simulink model "EngineDynamometer"  (R2025b)
settings: configuration reference "EngDynoVariable" (kept outside this file)
model workspace (MAT data in the model file):
  DynOperatingPts : timeseries (value not decoded)
undefined symbols (not defined in the file): CiDynoMaxTurboSpd, CiDynoSSSpdCmd, CiDynoSSTrqCmd, DynoResultsBlock, EnvAbsPrs, EnvAirTemp, EnvRair, ExhCamPhaseCmd, InjPw, IntkCamPhaseCmd, Line, PlntEngAfrStoich, PlntEngCps, PlntEngNCyl, PlntEngSinj, PlntEngVd, si, si0, SiDynoMaxTurboSpd, SiDynoOpenLoopEngSpdCmdPts, SiDynoOpenLoopExhCamPhsCmdPts, SiDynoOpenLoopIntCamPhsCmdPts, SiDynoOpenLoopLambdaCmdPts, SiDynoOpenLoopMaxMAP, SiDynoOpenLoopSpkDeltaCmdPts, SiDynoOpenLoopSteadyStateWaitLimit, SiDynoOpenLoopTpCmdPts, SiDynoOpenLoopWAPCmdPts, SiDynoSSSpdCmd, SiDynoSSTrqCmd, SiDynoSSWaitLim, SpkAdv, ThrPosPctCmd, WgAreaPctCmd
libraries: autolibutils x4, autolibpowerinfoutils x1, simulink x1
(part 2 of 3)

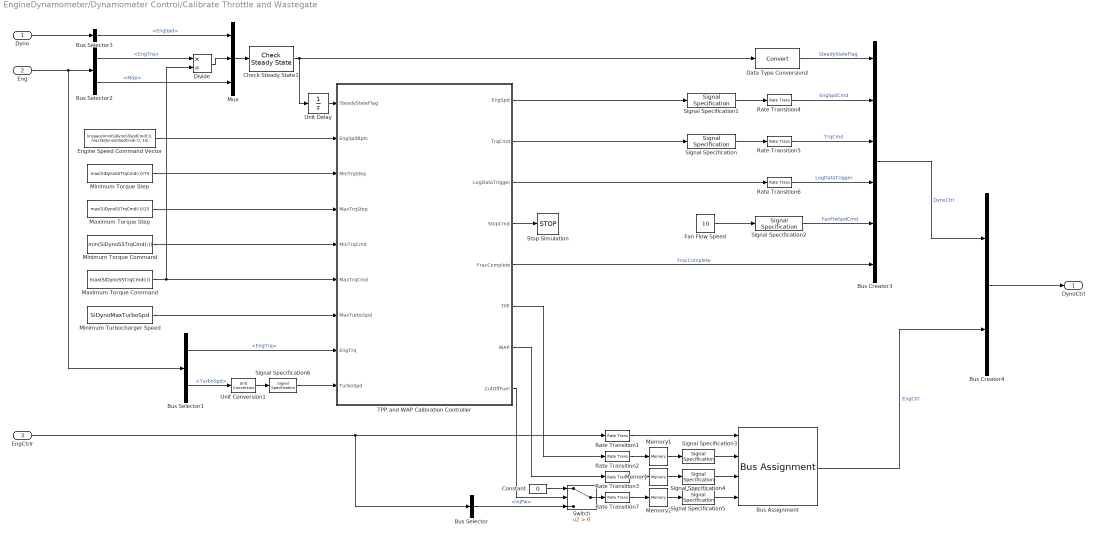
== system EngineDynamometer/Dynamometer Control/Calibrate Throttle and Wastegate ==
  Dyno : Inport
  Eng : Inport  Port=2
  EngCtrlr : Inport  Port=3
  Bus Assignment : BusAssignment  AssignedSignals=ThrPosPctCmd,WgAreaPctCmd,InjPw
  Bus Creator3 : BusCreator  Inputs=6
  Bus Creator4 : BusCreator  Inputs=2
  Bus Selector : BusSelector  OutputSignals=InjPw
  Bus Selector1 : BusSelector  OutputSignals=EngPlnt.EngTrq,EngPlnt.TurboSpd
  Bus Selector2 : BusSelector  OutputSignals=EngPlnt.EngTrq,EngPlnt.Map
  Bus Selector3 : BusSelector  OutputSignals=DynoPlnt.EngSpd
  Check Steady State1 : autolibutils/Check Steady State  N=4  F=50  Ts=0.2  SteadyThresh=[0.1; 0.003; 2500]  HoldTime=0.5  aMode=aMode
  Constant : Constant  Value=0
  Data Type Conversion2 : DataTypeConversion  SaturateOnIntegerOverflow=off  RndMeth=Floor
  Divide : Product  Inputs=*/
  Engine Speed Command Vector : Constant  Value=linspace(min(SiDynoSSSpdCmd(:)), max(SiDynoSSSpdCmd(:)), 15)
  Fan Flow Speed : Constant  Value=10
  Maximum Torque Command : Constant  Value=max(SiDynoSSTrqCmd(:))
  Maximum Torque Step : Constant  Value=max(SiDynoSSTrqCmd(:))/25
  Memory : Memory  InitialCondition=100
  Memory1 : Memory
  Memory2 : Memory  InitialCondition=100
  Minimum Torque Command : Constant  Value=min(SiDynoSSTrqCmd(:))
  Minimum Torque Step : Constant  Value=max(SiDynoSSTrqCmd(:))/75
  Minimum Turbocharger Speed : Constant  Value=SiDynoMaxTurboSpd
  Mux : Mux  Inputs=3
  Rate Transition{1..3,7} (4 alike) : RateTransition  Deterministic=off  OutPortSampleTimeOpt=Inherit
  Rate Transition4 : RateTransition  Deterministic=off
  Rate Transition5 : RateTransition  Deterministic=off
  Rate Transition6 : RateTransition  Deterministic=off
  Signal Specification : SignalSpecification  Unit=N*m
  Signal Specification1 : SignalSpecification  Unit=rpm
  Signal Specification2 : SignalSpecification  Unit=N*m
  Signal Specification3 : SignalSpecification  Unit=%
  Signal Specification4 : SignalSpecification  Unit=%
  Signal Specification5 : SignalSpecification  Unit=ms
  Signal Specification6 : SignalSpecification  Unit=rpm
  Stop Simulation : Stop
  Switch : Switch  Criteria=u2 > Threshold  SaturateOnIntegerOverflow=off  InputSameDT=off
  TPP and WAP Calibration Controller : Stateflow chart  TreatAsAtomicUnit=on
  Unit Conversion1 : UnitConversion
  Unit Delay : UnitDelay  SampleTime=-1  HasFrameUpgradeWarning=on
  DynoCtrl : Outport  VectorParamsAs1DForOutWhenUnconnected=off
  wires:
  Divide/1 -> Mux/2
  Bus Selector3/1 -> Mux/1  "<EngSpd>"
  Bus Selector2/1 -> Divide/1  "<EngTrq>"
  TPP and WAP Calibration Controller/2(TrqCmd) -> Signal Specification/1
  Bus Selector2/2 -> Mux/3  "<Map>"
  TPP and WAP Calibration Controller/7(WAP) -> Rate Transition3/1
  TPP and WAP Calibration Controller/6(TPP) -> Rate Transition2/1
  Bus Creator3/1 -> Bus Creator4/1  "DynoCtrl"
  Bus Creator4/1 -> DynoCtrl/1
  Mux/1 -> Check Steady State1/1
  Data Type Conversion2/1 -> Bus Creator3/1  "SteadyStateFlag"
  Rate Transition6/1 -> Bus Creator3/4  "LogDataTrigger"
  Rate Transition5/1 -> Bus Creator3/3  "TrqCmd"
  Rate Transition4/1 -> Bus Creator3/2  "EngSpdCmd"
  Fan Flow Speed/1 -> Signal Specification2/1
  Maximum Torque Step/1 -> TPP and WAP Calibration Controller/4(MaxTrqStep)
  Engine Speed Command Vector/1 -> TPP and WAP Calibration Controller/2(EngSpdBpts)
  TPP and WAP Calibration Controller/4(StopCmd) -> Stop Simulation/1
  Dyno/1 -> Bus Selector3/1
  Eng/1 -> Bus Selector1/1, Bus Selector2/1
  Rate Transition3/1 -> Memory/1
  Rate Transition2/1 -> Memory1/1
  Bus Selector1/1 -> TPP and WAP Calibration Controller/8(EngTrq)  "<EngTrq>"
  Bus Selector1/2 -> Unit Conversion1/1  "<TurboSpd>"
  Signal Specification/1 -> Rate Transition5/1
  Signal Specification1/1 -> Rate Transition4/1
  TPP and WAP Calibration Controller/1(EngSpd) -> Signal Specification1/1
  Signal Specification2/1 -> Bus Creator3/5  "FanFlwSpdCmd"
  TPP and WAP Calibration Controller/5(FracComplete) -> Bus Creator3/6  "FracComplete"
  EngCtrlr/1 -> Rate Transition1/1, Bus Selector/1
  Memory/1 -> Signal Specification4/1
  Memory1/1 -> Signal Specification3/1
  Bus Assignment/1 -> Bus Creator4/2  "EngCtrl"
  Signal Specification3/1 -> Bus Assignment/2
  Signal Specification4/1 -> Bus Assignment/3
  Rate Transition1/1 -> Bus Assignment/1
  Minimum Torque Step/1 -> TPP and WAP Calibration Controller/3(MinTrqStep)
  Minimum Torque Command/1 -> TPP and WAP Calibration Controller/5(MinTrqCmd)
  Maximum Torque Command/1 -> Divide/2, TPP and WAP Calibration Controller/6(MaxTrqCmd)
  Check Steady State1/1 -> Unit Delay/1, Data Type Conversion2/1
  TPP and WAP Calibration Controller/3(LogDataTrigger) -> Rate Transition6/1
  Minimum Turbocharger Speed/1 -> TPP and WAP Calibration Controller/7(MaxTurboSpd)
  Unit Conversion1/1 -> Signal Specification6/1
  Signal Specification6/1 -> TPP and WAP Calibration Controller/9(TurboSpd)
  Memory2/1 -> Signal Specification5/1
  Rate Transition7/1 -> Memory2/1
  Signal Specification5/1 -> Bus Assignment/4
  Switch/1 -> Rate Transition7/1
  TPP and WAP Calibration Controller/8(CutOffFuel) -> Switch/2
  Constant/1 -> Switch/1
  Bus Selector/1 -> Switch/3  "<InjPw>"
  Unit Delay/1 -> TPP and WAP Calibration Controller/1(SteadyStateFlag)

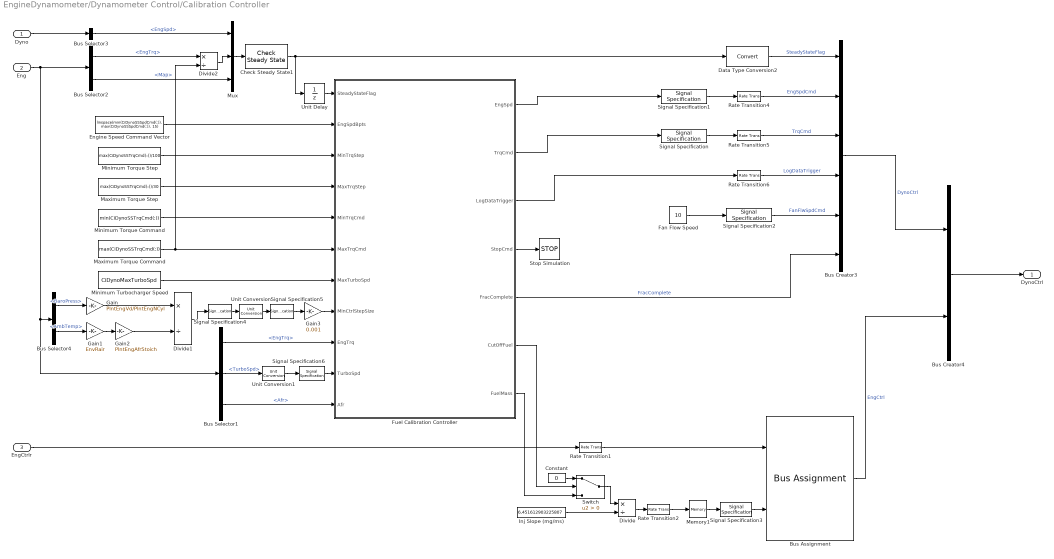
== system EngineDynamometer/Dynamometer Control/Calibration Controller ==
  Dyno : Inport
  Eng : Inport  Port=2
  EngCtrlr : Inport  Port=3
  Bus Assignment : BusAssignment  AssignedSignals=InjPw
  Bus Creator3 : BusCreator  Inputs=6
  Bus Creator4 : BusCreator  Inputs=2
  Bus Selector1 : BusSelector  OutputSignals=EngPlnt.EngTrq,EngPlnt.TurboSpd,EngPlnt.Afr
  Bus Selector2 : BusSelector  OutputSignals=EngPlnt.EngTrq,EngPlnt.Map
  Bus Selector3 : BusSelector  OutputSignals=DynoPlnt.EngSpd
  Bus Selector4 : BusSelector  OutputSignals=Env.BaroPress,Env.AmbTemp
  Check Steady State1 : autolibutils/Check Steady State  N=4  F=25  Ts=0.1  SteadyThresh=[0.1; 0.002; 500]  HoldTime=0.5  aMode=aMode
  Constant : Constant  Value=0
  Data Type Conversion2 : DataTypeConversion  SaturateOnIntegerOverflow=off  RndMeth=Floor
  Divide : Product  Inputs=*/
  Divide1 : Product  Inputs=*/
  Divide2 : Product  Inputs=*/
  Engine Speed Command Vector : Constant  Value=linspace(min(CiDynoSSSpdCmd(:)), max(CiDynoSSSpdCmd(:)), 15)
  Fan Flow Speed : Constant  Value=10
  Fuel Calibration Controller : Stateflow chart  TreatAsAtomicUnit=on
  Gain : Gain  Gain=PlntEngVd/PlntEngNCyl
  Gain1 : Gain  Gain=EnvRair
  Gain2 : Gain  Gain=PlntEngAfrStoich
  Gain3 : Gain  Gain=0.001
  Inj Slope (mg/ms) : Constant  Value=6.451612903225807
  Maximum Torque Command : Constant  Value=max(CiDynoSSTrqCmd(:))
  Maximum Torque Step : Constant  Value=max(CiDynoSSTrqCmd(:))/30
  Memory1 : Memory
  Minimum Torque Command : Constant  Value=min(CiDynoSSTrqCmd(:))
  Minimum Torque Step : Constant  Value=max(CiDynoSSTrqCmd(:))/100
  Minimum Turbocharger Speed : Constant  Value=CiDynoMaxTurboSpd
  Mux : Mux  Inputs=3
  Rate Transition1 : RateTransition  Deterministic=off  OutPortSampleTimeOpt=Inherit
  Rate Transition2 : RateTransition  Deterministic=off  OutPortSampleTimeOpt=Inherit
  Rate Transition4 : RateTransition  Deterministic=off
  Rate Transition5 : RateTransition  Deterministic=off
  Rate Transition6 : RateTransition  Deterministic=off
  Signal Specification : SignalSpecification  Unit=N*m
  Signal Specification1 : SignalSpecification  Unit=rpm
  Signal Specification2 : SignalSpecification  Unit=N*m
  Signal Specification3 : SignalSpecification  Unit=ms
  Signal Specification4 : SignalSpecification  Unit=kg
  Signal Specification5 : SignalSpecification  Unit=mg
  Signal Specification6 : SignalSpecification  Unit=rpm
  Stop Simulation : Stop
  Switch : Switch  Criteria=u2 > Threshold  SaturateOnIntegerOverflow=off  InputSameDT=off
  Unit Conversion : UnitConversion
  Unit Conversion1 : UnitConversion
  Unit Delay : UnitDelay  SampleTime=-1  HasFrameUpgradeWarning=on
  DynoCtrl : Outport  VectorParamsAs1DForOutWhenUnconnected=off
  wires:
  Signal Specification5/1 -> Gain3/1
  Gain3/1 -> Fuel Calibration Controller/8(MinCtrlStepSize)
  Unit Conversion/1 -> Signal Specification5/1
  Divide1/1 -> Signal Specification4/1
  Signal Specification4/1 -> Unit Conversion/1
  Gain2/1 -> Divide1/2
  Gain/1 -> Divide1/1
  Gain1/1 -> Gain2/1
  Bus Selector4/1 -> Gain/1  "<BaroPress>"
  Bus Selector4/2 -> Gain1/1  "<AmbTemp>"
  Bus Selector3/1 -> Mux/1  "<EngSpd>"
  Bus Selector2/1 -> Divide2/1  "<EngTrq>"
  Fuel Calibration Controller/2(TrqCmd) -> Signal Specification/1
  Bus Selector2/2 -> Mux/3  "<Map>"
  Bus Creator3/1 -> Bus Creator4/1  "DynoCtrl"
  Bus Creator4/1 -> DynoCtrl/1
  Mux/1 -> Check Steady State1/1
  Data Type Conversion2/1 -> Bus Creator3/1  "SteadyStateFlag"
  Rate Transition6/1 -> Bus Creator3/4  "LogDataTrigger"
  Rate Transition5/1 -> Bus Creator3/3  "TrqCmd"
  Rate Transition4/1 -> Bus Creator3/2  "EngSpdCmd"
  Fan Flow Speed/1 -> Signal Specification2/1
  Maximum Torque Step/1 -> Fuel Calibration Controller/4(MaxTrqStep)
  Engine Speed Command Vector/1 -> Fuel Calibration Controller/2(EngSpdBpts)
  Fuel Calibration Controller/4(StopCmd) -> Stop Simulation/1
  Dyno/1 -> Bus Selector3/1
  Eng/1 -> Bus Selector4/1, Bus Selector1/1, Bus Selector2/1
  Rate Transition2/1 -> Memory1/1
  Bus Selector1/1 -> Fuel Calibration Controller/9(EngTrq)  "<EngTrq>"
  Bus Selector1/2 -> Unit Conversion1/1  "<TurboSpd>"
  Signal Specification/1 -> Rate Transition5/1
  Signal Specification1/1 -> Rate Transition4/1
  Fuel Calibration Controller/1(EngSpd) -> Signal Specification1/1
  Signal Specification2/1 -> Bus Creator3/5  "FanFlwSpdCmd"
  Fuel Calibration Controller/5(FracComplete) -> Bus Creator3/6  "FracComplete"
  EngCtrlr/1 -> Rate Transition1/1
  Memory1/1 -> Signal Specification3/1
  Bus Assignment/1 -> Bus Creator4/2  "EngCtrl"
  Signal Specification3/1 -> Bus Assignment/2
  Rate Transition1/1 -> Bus Assignment/1
  Minimum Torque Step/1 -> Fuel Calibration Controller/3(MinTrqStep)
  Minimum Torque Command/1 -> Fuel Calibration Controller/5(MinTrqCmd)
  Check Steady State1/1 -> Data Type Conversion2/1, Unit Delay/1
  Fuel Calibration Controller/3(LogDataTrigger) -> Rate Transition6/1
  Bus Selector1/3 -> Fuel Calibration Controller/11(Afr)  "<Afr>"
  Inj Slope (mg/ms)/1 -> Divide/2
  Divide/1 -> Rate Transition2/1
  Divide2/1 -> Mux/2
  Maximum Torque Command/1 -> Fuel Calibration Controller/6(MaxTrqCmd), Divide2/2
  Minimum Turbocharger Speed/1 -> Fuel Calibration Controller/7(MaxTurboSpd)
  Unit Conversion1/1 -> Signal Specification6/1
  Signal Specification6/1 -> Fuel Calibration Controller/10(TurboSpd)
  Constant/1 -> Switch/1
  Fuel Calibration Controller/6(CutOffFuel) -> Switch/2
  Switch/1 -> Divide/1
  Fuel Calibration Controller/7(FuelMass) -> Switch/3
  Unit Delay/1 -> Fuel Calibration Controller/1(SteadyStateFlag)

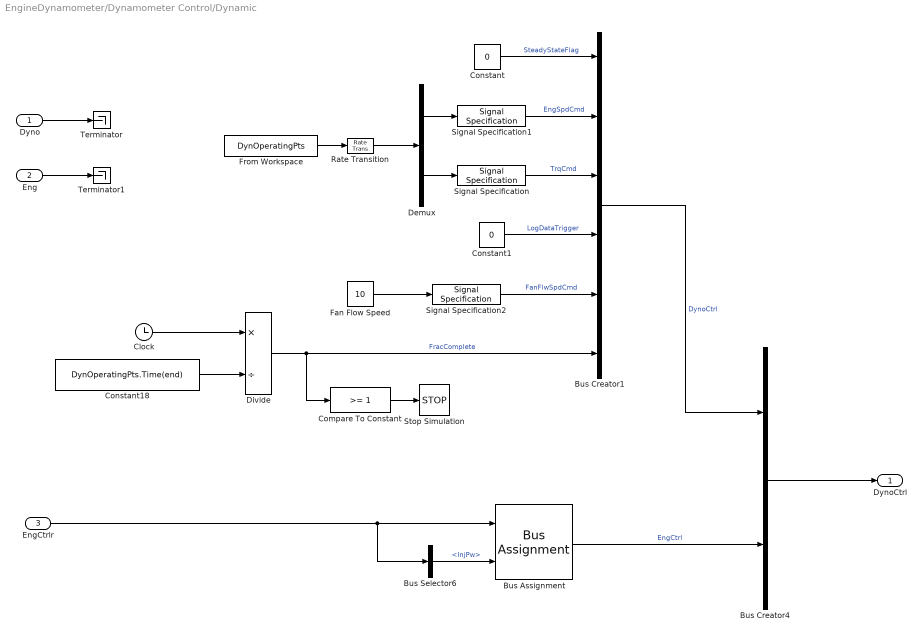
== system EngineDynamometer/Dynamometer Control/Dynamic ==
  Dyno : Inport
  Eng : Inport  Port=2
  EngCtrlr : Inport  Port=3
  Bus Assignment : BusAssignment  AssignedSignals=InjPw
  Bus Creator1 : BusCreator  Inputs=6
  Bus Creator4 : BusCreator  Inputs=2
  Bus Selector6 : BusSelector  OutputSignals=InjPw
  Clock : Clock
  Compare To Constant : simulink/Logic and Bit Operations/Compare To Constant  relop=>=  const=1  OutDataTypeStr=boolean
  Constant : Constant  Value=0
  Constant1 : Constant  Value=0
  Constant18 : Constant  Value=DynOperatingPts.Time(end)
  Demux : Demux  Outputs=2
  Divide : Product  Inputs=*/
  Fan Flow Speed : Constant  Value=10
  From Workspace : FromWorkspace  VariableName=DynOperatingPts  SampleTime=0.01  ZeroCross=off  OutputAfterFinalValue=Holding final value
  Rate Transition : RateTransition
  Signal Specification : SignalSpecification  Unit=N*m
  Signal Specification1 : SignalSpecification  Unit=rpm
  Signal Specification2 : SignalSpecification  Unit=m/s
  Stop Simulation : Stop
  Terminator : Terminator
  Terminator1 : Terminator
  DynoCtrl : Outport  VectorParamsAs1DForOutWhenUnconnected=off
  wires:
  Bus Creator1/1 -> Bus Creator4/1  "DynoCtrl"
  Bus Creator4/1 -> DynoCtrl/1
  Constant1/1 -> Bus Creator1/4  "LogDataTrigger"
  Constant/1 -> Bus Creator1/1  "SteadyStateFlag"
  Dyno/1 -> Terminator/1
  Demux/1 -> Signal Specification1/1
  Demux/2 -> Signal Specification/1
  Clock/1 -> Divide/1
  Compare To Constant/1 -> Stop Simulation/1
  From Workspace/1 -> Rate Transition/1
  Rate Transition/1 -> Demux/1
  Fan Flow Speed/1 -> Signal Specification2/1
  Signal Specification2/1 -> Bus Creator1/5  "FanFlwSpdCmd"
  Signal Specification1/1 -> Bus Creator1/2  "EngSpdCmd"
  Signal Specification/1 -> Bus Creator1/3  "TrqCmd"
  Divide/1 -> Compare To Constant/1, Bus Creator1/6  "FracComplete"
  Constant18/1 -> Divide/2
  EngCtrlr/1 -> Bus Assignment/1, Bus Selector6/1
  Bus Assignment/1 -> Bus Creator4/2  "EngCtrl"
  Bus Selector6/1 -> Bus Assignment/2  "<InjPw>"
  Eng/1 -> Terminator1/1

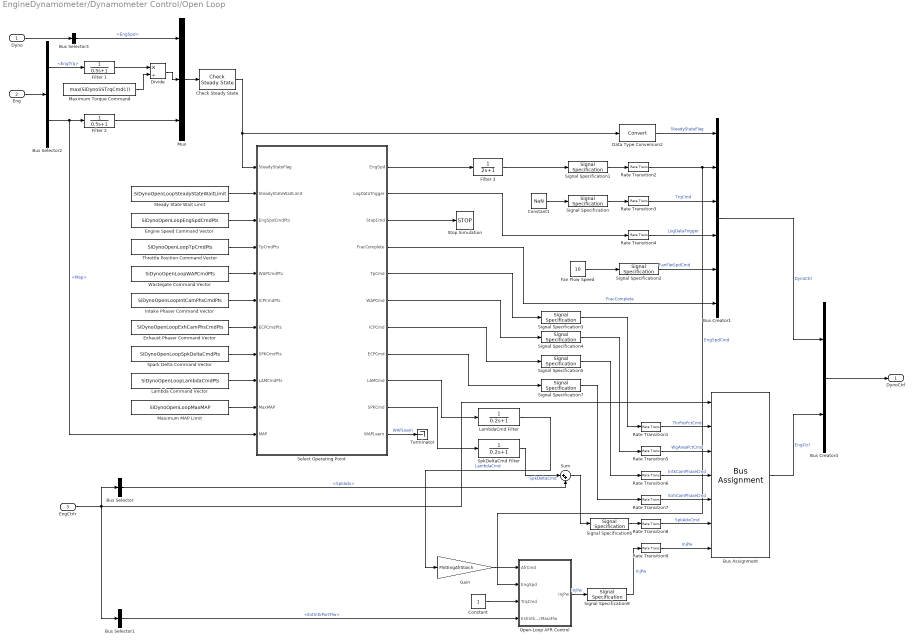
== system EngineDynamometer/Dynamometer Control/Open Loop ==
  Dyno : Inport
  Eng : Inport  Port=2
  EngCtrlr : Inport  Port=3
  Bus Assignment : BusAssignment  AssignedSignals=ThrPosPctCmd,WgAreaPctCmd,IntkCamPhaseCmd,ExhCamPhaseCmd,SpkAdv,InjPw
  Bus Creator1 : BusCreator  Inputs=6
  Bus Creator4 : BusCreator  Inputs=2
  Bus Selector : BusSelector  OutputSignals=SpkAdv
  Bus Selector1 : BusSelector  OutputSignals=EstIntkPortFlw
  Bus Selector2 : BusSelector  OutputSignals=EngPlnt.EngTrq,EngPlnt.Map
  Bus Selector3 : BusSelector  OutputSignals=DynoPlnt.EngSpd
  Check Steady State : autolibutils/Check Steady State  N=4  F=25  Ts=0.1  SteadyThresh=[0.25; 0.002; 2000]  HoldTime=1  aMode=aMode
  Constant : Constant
  Constant1 : Constant  Value=NaN
  Data Type Conversion2 : DataTypeConversion  SaturateOnIntegerOverflow=off  RndMeth=Floor
  Divide : Product  Inputs=*/
  Engine Speed Command Vector : Constant  Value=SiDynoOpenLoopEngSpdCmdPts
  Exhaust Phaser Command Vector : Constant  Value=SiDynoOpenLoopExhCamPhsCmdPts
  Fan Flow Speed : Constant  Value=10
  Filter 1 : TransferFcn  Denominator=[0.5 1]
  Filter 2 : TransferFcn  Denominator=[0.5 1]
  Filter 3 : TransferFcn  Denominator=[2 1]
  Gain : Gain  Gain=PlntEngAfrStoich
  Intake Phaser Command Vector : Constant  Value=SiDynoOpenLoopIntCamPhsCmdPts
  Lambda Command Vector : Constant  Value=SiDynoOpenLoopLambdaCmdPts
  LambdaCmd Filter : TransferFcn  Denominator=[0.2 1]
  Maximum MAP Limit : Constant  Value=SiDynoOpenLoopMaxMAP
  Maximum Torque Command : Constant  Value=max(SiDynoSSTrqCmd(:))
  Mux : Mux  Inputs=3
  Open-Loop AFR Control : Subsystem
      settings: LibrarySourceBlock=autolibengctrlr/SI Controller/Controllers/Fuel/Open-Loop AFR Control
  Rate Transition{1..9} (9 alike) : RateTransition
  Select Operating Point : Stateflow chart  TreatAsAtomicUnit=on
      settings: PortSchema="{\"entries\":[{\"content\":{\"sides\":[{\"content\":{\"connectorIds\":[\"In1\",\"In2\",\"In3\",\"In4\",\"In5\",\"In6\",\"In7\",\"In8\",\"In9\",\"In11\",\"In10\"]},\"type\":\"ConnectorPlacement.EquallySpacedRectSide\",\"uuid\":\"1175ad6d-9dc6-48de-a8de-c94bf62b3e4b\"},{\"content\":{\"connectorIds\":[\"Out1\",\"Out2\",\"Out3\",\"Out4\",\"Out5\",\"Out6\",\"Out7\",\"Out8\",\"Out9\",\"Out10\",\"Out11\"],\"side\":\"RIGHT\"},\"type\":\"ConnectorPlacement.EquallySpacedRectSide\",\"uuid\":\"1be9bb31-04dd-492d-b81f-3e8c0fe512b8\"},{\"content\":{\"connectorIds\":[],\"side\":\"TOP\"},\"type\":\"ConnectorPlacement.EquallySpacedRectSide\",\"uuid\":\"9ff59bc2-c566-4c7d-a042-0eeecf9e5d1c\"}]},\"type\":\"ConnectorPlacement.EquallySpacedConnector\",\"uuid\":\"78b64ed8-c9b9-4ccc-b3ba-c3246a70f380\"}],\"packageUris\":[\"http://schema.mathworks.com/mf0/Connector/R2020b\"],\"version\":\"1.0\"}"
  Signal Specification : SignalSpecification  Unit=N*m
  Signal Specification1 : SignalSpecification  Unit=rpm
  Signal Specification2 : SignalSpecification  Unit=m/s
  Signal Specification3 : SignalSpecification  Unit=%
  Signal Specification4 : SignalSpecification  Unit=%
  Signal Specification5 : SignalSpecification  Unit=deg
  Signal Specification6 : SignalSpecification  Unit=deg
  Signal Specification7 : SignalSpecification  Unit=deg
  Signal Specification8 : SignalSpecification  Unit=ms
  Spark Delta Command Vector : Constant  Value=SiDynoOpenLoopSpkDeltaCmdPts
  SpkDeltaCmd Filter : TransferFcn  Denominator=[0.2 1]
  Steady State Wait Limit : Constant  Value=SiDynoOpenLoopSteadyStateWaitLimit
  Stop Simulation : Stop
  Sum : Sum  Inputs=|++
  Terminator : Terminator
  Throttle Position Command Vector : Constant  Value=SiDynoOpenLoopTpCmdPts
  Wastegate Command Vector : Constant  Value=SiDynoOpenLoopWAPCmdPts
  DynoCtrl : Outport  VectorParamsAs1DForOutWhenUnconnected=off
  wires:
  Maximum Torque Command/1 -> Divide/2
  Divide/1 -> Mux/2
  Select Operating Point/4(FracComplete) -> Bus Creator1/6  "FracComplete"
  Signal Specification/1 -> Rate Transition3/1
  Signal Specification1/1 -> Rate Transition2/1
  Signal Specification2/1 -> Bus Creator1/5  "FanFlwSpdCmd"
  Fan Flow Speed/1 -> Signal Specification2/1
  Engine Speed Command Vector/1 -> Select Operating Point/3(EngSpdCmdPts)
  Throttle Position Command Vector/1 -> Select Operating Point/4(TpCmdPts)
  Select Operating Point/2(LogDataTrigger) -> Rate Transition4/1
  Rate Transition2/1 -> Open-Loop AFR Control/2(EngSpd), Bus Creator1/2  "EngSpdCmd"
  Rate Transition3/1 -> Bus Creator1/3  "TrqCmd"
  Rate Transition4/1 -> Bus Creator1/4  "LogDataTrigger"
  Data Type Conversion2/1 -> Bus Creator1/1  "SteadyStateFlag"
  Check Steady State/1 -> Data Type Conversion2/1, Select Operating Point/1(SteadyStateFlag)
  Bus Creator4/1 -> DynoCtrl/1
  Bus Creator1/1 -> Bus Creator4/1  "DynoCtrl"
  Bus Assignment/1 -> Bus Creator4/2  "EngCtrl"
  Eng/1 -> Bus Selector2/1
  Dyno/1 -> Bus Selector3/1
  Mux/1 -> Check Steady State/1
  Bus Selector3/1 -> Mux/1  "<EngSpd>"
  EngCtrlr/1 -> Bus Selector1/1, Bus Selector/1, Bus Assignment/1
  Steady State Wait Limit/1 -> Select Operating Point/2(SteadyStateWaitLimit)
  Bus Selector2/1 -> Filter 1/1  "<EngTrq>"
  Filter 1/1 -> Divide/1
  Bus Selector2/2 -> Select Operating Point/10(MAP), Filter 2/1  "<Map>"
  Filter 2/1 -> Mux/3
  Filter 3/1 -> Signal Specification1/1
  Wastegate Command Vector/1 -> Select Operating Point/5(WAPCmdPts)
  Rate Transition1/1 -> Bus Assignment/2  "ThrPosPctCmd"
  Select Operating Point/5(TpCmd) -> Signal Specification3/1
  Select Operating Point/6(WAPCmd) -> Signal Specification4/1
  Rate Transition5/1 -> Bus Assignment/3  "WgAreaPctCmd"
  Select Operating Point/1(EngSpd) -> Filter 3/1
  Select Operating Point/3(StopCmd) -> Stop Simulation/1
  Intake Phaser Command Vector/1 -> Select Operating Point/6(ICPCmdPts)
  Exhaust Phaser Command Vector/1 -> Select Operating Point/7(ECPCmdPts)
  Signal Specification5/1 -> Rate Transition6/1
  Signal Specification7/1 -> Rate Transition7/1
  Select Operating Point/7(ICPCmd) -> Signal Specification5/1
  Select Operating Point/8(ECPCmd) -> Signal Specification7/1
  Rate Transition7/1 -> Bus Assignment/5  "ExhCamPhaseCmd"
  Rate Transition6/1 -> Bus Assignment/4  "IntkCamPhaseCmd"
  Spark Delta Command Vector/1 -> Select Operating Point/8(SPKCmdPts)
  Lambda Command Vector/1 -> Select Operating Point/9(LAMCmdPts)
  Select Operating Point/9(LAMCmd) -> LambdaCmd Filter/1
  Bus Selector/1 -> Sum/2  "<SpkAdv>"
  Sum/1 -> Signal Specification6/1
  Rate Transition8/1 -> Bus Assignment/6  "SpkAdvCmd"
  Signal Specification6/1 -> Rate Transition8/1
  LambdaCmd Filter/1 -> Gain/1  "LambdaCmd"
  SpkDeltaCmd Filter/1 -> Sum/1  "SpkDeltaCmd"
  Select Operating Point/10(SPKCmd) -> SpkDeltaCmd Filter/1
  Gain/1 -> Open-Loop AFR Control/1(AfrCmd)
  Constant/1 -> Open-Loop AFR Control/3(TrqCmd)
  Rate Transition9/1 -> Bus Assignment/7  "InjPw"
  Open-Loop AFR Control/1(InjPw) -> Signal Specification8/1  "InjPw"
  Signal Specification8/1 -> Rate Transition9/1  "InjPw"
  Bus Selector1/1 -> Open-Loop AFR Control/4(EstIntkAirMassFlw)  "<EstIntkPortFlw>"
  Signal Specification3/1 -> Rate Transition1/1
  Signal Specification4/1 -> Rate Transition5/1
  Maximum MAP Limit/1 -> Select Operating Point/11(MaxMAP)
  Select Operating Point/11(WAPLearn) -> Terminator/1  "WAPLearn"
  Constant1/1 -> Signal Specification/1

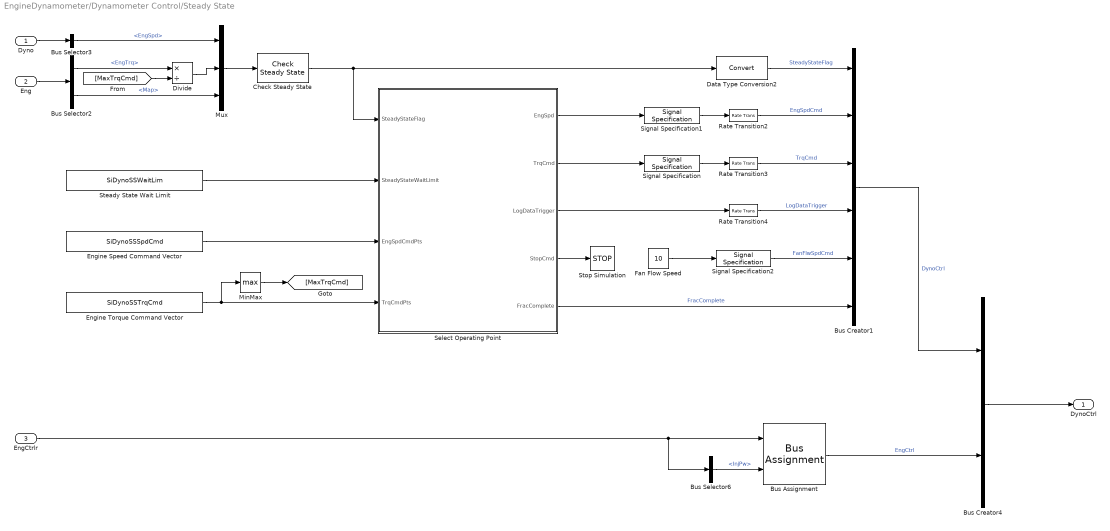
== system EngineDynamometer/Dynamometer Control/Steady State ==
  Dyno : Inport
  Eng : Inport  Port=2
  EngCtrlr : Inport  Port=3
  Bus Assignment : BusAssignment  AssignedSignals=InjPw
  Bus Creator1 : BusCreator  Inputs=6
  Bus Creator4 : BusCreator  Inputs=2
  Bus Selector2 : BusSelector  OutputSignals=EngPlnt.EngTrq,EngPlnt.Map
  Bus Selector3 : BusSelector  OutputSignals=DynoPlnt.EngSpd
  Bus Selector6 : BusSelector  OutputSignals=InjPw
  Check Steady State : autolibutils/Check Steady State  N=4  F=25  Ts=0.1  SteadyThresh=[0.25; 0.002; 2000]  HoldTime=1  aMode=aMode
  Data Type Conversion2 : DataTypeConversion  SaturateOnIntegerOverflow=off  RndMeth=Floor
  Divide : Product  Inputs=*/
  Engine Speed Command Vector : Constant  Value=SiDynoSSSpdCmd
  Engine Torque Command Vector : Constant  Value=SiDynoSSTrqCmd
  Fan Flow Speed : Constant  Value=10
  MinMax : MinMax  Function=max
  Mux : Mux  Inputs=3
  Rate Transition2 : RateTransition
  Rate Transition3 : RateTransition
  Rate Transition4 : RateTransition
  Select Operating Point : Stateflow chart  TreatAsAtomicUnit=on
  Signal Specification : SignalSpecification  Unit=N*m
  Signal Specification1 : SignalSpecification  Unit=rpm
  Signal Specification2 : SignalSpecification  Unit=m/s
  Steady State Wait Limit : Constant  Value=SiDynoSSWaitLim
  Stop Simulation : Stop
  DynoCtrl : Outport  VectorParamsAs1DForOutWhenUnconnected=off
  wires:
  Divide/1 -> Mux/2
  Select Operating Point/5(FracComplete) -> Bus Creator1/6  "FracComplete"
  Signal Specification/1 -> Rate Transition3/1
  Signal Specification1/1 -> Rate Transition2/1
  Signal Specification2/1 -> Bus Creator1/5  "FanFlwSpdCmd"
  Fan Flow Speed/1 -> Signal Specification2/1
  Select Operating Point/4(StopCmd) -> Stop Simulation/1
  Engine Speed Command Vector/1 -> Select Operating Point/3(EngSpdCmdPts)
  Engine Torque Command Vector/1 -> MinMax/1, Select Operating Point/4(TrqCmdPts)
  Select Operating Point/1(EngSpd) -> Signal Specification1/1
  Select Operating Point/2(TrqCmd) -> Signal Specification/1
  Select Operating Point/3(LogDataTrigger) -> Rate Transition4/1
  Rate Transition2/1 -> Bus Creator1/2  "EngSpdCmd"
  Rate Transition3/1 -> Bus Creator1/3  "TrqCmd"
  Rate Transition4/1 -> Bus Creator1/4  "LogDataTrigger"
  Data Type Conversion2/1 -> Bus Creator1/1  "SteadyStateFlag"
  Check Steady State/1 -> Select Operating Point/1(SteadyStateFlag), Data Type Conversion2/1
  Bus Creator4/1 -> DynoCtrl/1
  Bus Creator1/1 -> Bus Creator4/1  "DynoCtrl"
  Bus Assignment/1 -> Bus Creator4/2  "EngCtrl"
  Eng/1 -> Bus Selector2/1
  Dyno/1 -> Bus Selector3/1
  Mux/1 -> Check Steady State/1
  Bus Selector2/2 -> Mux/3  "<Map>"
  Bus Selector2/1 -> Divide/1  "<EngTrq>"
  Bus Selector3/1 -> Mux/1  "<EngSpd>"
  EngCtrlr/1 -> Bus Selector6/1, Bus Assignment/1
  Bus Selector6/1 -> Bus Assignment/2  "<InjPw>"
  Steady State Wait Limit/1 -> Select Operating Point/2(SteadyStateWaitLimit)
  MinMax/1 -> [MaxTrqCmd]
  [MaxTrqCmd] -> Divide/2

== system EngineDynamometer/Engine System/Dynamometer Engine Control ==
  Dyno : Inport
  Bus Selector : BusSelector  OutputSignals=DynoCtrl.EngCtrl
  Ctrl : Outport  VectorParamsAs1DForOutWhenUnconnected=off
  wires:
  Dyno/1 -> Bus Selector/1
  Bus Selector/1 -> Ctrl/1  "<EngCtrl>"

== system EngineDynamometer/Engine System/Engine Controller ==
  Env : Inport
  Dyno : Inport  Port=2
  EngPlnt : Inport  Port=3
  Engine Control : Subsystem  Variant=on  VariantControlMode=label  VariantControl=Choice  LabelModeActiveChoice=SI Engine Controller
  Engine Control Input : Subsystem
  Engine Control Output : Subsystem
  EngCtrlrOutput : Outport  VectorParamsAs1DForOutWhenUnconnected=off
  wires:
  Engine Control Output/1(EngCtrlrOutput) -> EngCtrlrOutput/1
  Dyno/1 -> Engine Control Input/1(Dyno)
  Env/1 -> Engine Control Input/2(Env)
  EngPlnt/1 -> Engine Control Input/3(VehPlnt)
  Engine Control Input/1(TrqCmd) -> Engine Control/1(TrqCmd)
  Engine Control Input/2(EngSpd) -> Engine Control/2(EngSpd)
  Engine Control Input/3(Map) -> Engine Control/3(Map)
  Engine Control Input/4(Mat) -> Engine Control/4(Mat)
  Engine Control Input/5(ThrPosPct) -> Engine Control/5(ThrPosPct)
  Engine Control Input/6(WgAreaPct) -> Engine Control/6(WgAreaPct)
  Engine Control Input/7(IntkCamPhase) -> Engine Control/7(IntkCamPhase)
  Engine Control Input/8(ExhCamPhase) -> Engine Control/8(ExhCamPhase)
  Engine Control Input/9(TurboRackPos) -> Engine Control/9(TurboRackPos)
  Engine Control Input/10(EgrVlvAreaPct) -> Engine Control/10(EgrVlvAreaPct)
  Engine Control Input/11(VarCompRatioPos) -> Engine Control/11(VarCompRatioPos)
  Engine Control Input/12(IntkVlvLift) -> Engine Control/12(IntkVlvLift)
  Engine Control Input/13(VarIntkRunLen) -> Engine Control/13(VarIntkRunLen)
  Engine Control Input/14(Afr) -> Engine Control/14(Afr)
  Engine Control Input/15(IntkSwirlVlvPos) -> Engine Control/15(IntkSwirlVlvPos)
  Engine Control Input/16(TurboSpd) -> Engine Control/16(TurboSpd)
  Engine Control Input/17(AmbPrs) -> Engine Control/17(AmbPrs)
  Engine Control Input/18(IgSw) -> Engine Control/18(IgSw)
  Engine Control Input/19(Iat) -> Engine Control/19(Iat)
  Engine Control Input/20(Ect) -> Engine Control/20(Ect)
  Engine Control Input/21(EgrVlvDeltaPrs) -> Engine Control/21(EgrVlvDeltaPrs)
  Engine Control Input/22(EgrVlvInTemp) -> Engine Control/22(EgrVlvInTemp)
  Engine Control/1(ThrPosPctCmd) -> Engine Control Output/1(ThrPosPctCmd)
  Engine Control/2(WgAreaPctCmd) -> Engine Control Output/2(WgAreaPctCmd)
  Engine Control/3(InjPw) -> Engine Control Output/3(InjPw)
  Engine Control/4(FuelMainSoi) -> Engine Control Output/4(FuelMainSoi)
  Engine Control/5(SpkAdv) -> Engine Control Output/5(SpkAdv)
  Engine Control/6(IntkCamPhaseCmd) -> Engine Control Output/6(IntkCamPhaseCmd)
  Engine Control/7(ExhCamPhaseCmd) -> Engine Control Output/7(ExhCamPhaseCmd)
  Engine Control/8(TurboRackPosCmd) -> Engine Control Output/8(TurboRackPosCmd)
  Engine Control/9(EgrVlvAreaPctCmd) -> Engine Control Output/9(EgrVlvAreaPctCmd)
  Engine Control/10(VarCompRatioPosCmd) -> Engine Control Output/10(VarCompRatioPosCmd)
  Engine Control/11(IntkVlvLiftCmd) -> Engine Control Output/11(IntkVlvLiftCmd)
  Engine Control/12(VarIntkRunLenCmd) -> Engine Control Output/12(VarIntkRunLenCmd)
  Engine Control/13(ClsdLpFuelMult) -> Engine Control Output/13(ClsdLpFuelMult)
  Engine Control/14(IntkSwirlVlvPosCmd) -> Engine Control Output/14(IntkSwirlVlvPosCmd)
  Engine Control/15(TrqCmdISC) -> Engine Control Output/15(TrqCmdISC)
  Engine Control/16(LoadCmd) -> Engine Control Output/16(LoadCmd)
  Engine Control/17(EstIntkPortFlw) -> Engine Control Output/17(EstIntkPortFlw)

== system EngineDynamometer/Engine System/Engine Plant ==
  Env : Inport
  Ctrl : Inport  Port=2
  Bus Element In1 : Inport  Port=3  PortName=Dyno  Element=DynoPlnt.FanFlwSpd
  Bus Element In3 : Inport  Port=3  PortName=Dyno  Element=DynoPlnt.EngSpd
  Engine : Subsystem  Variant=on  VariantControlMode=label  LabelModeActiveChoice=SI Engine
  Engine Plant Input : Subsystem
  EngFdbk : Outport
  wires:
  Env/1 -> Engine Plant Input/1(Env)
  Engine Plant Input/3(Dyno) -> Engine/3(Veh)
  Engine/1(EngFdbk) -> EngFdbk/1
  Engine Plant Input/1(EnvOut) -> Engine/1(Env)
  Engine Plant Input/2(EngineSpeed) -> Engine/2(EngSpd)
  Bus Element In3/1 -> Engine Plant Input/3(EngSpd)
  Bus Element In1/1 -> Engine Plant Input/4(Veh)
  Engine Plant Input/4(Ctrl) -> Engine/4(Cntrl)
  Ctrl/1 -> Engine Plant Input/2(Cntrl)

== system EngineDynamometer/Performance Monitor/CheckToStop ==
  <TrqCmd> : Inport
  <EngTrq> : Inport  Port=2
  Chart : Stateflow chart  TreatAsAtomicUnit=on
      settings: PortSchema="{\"entries\":[{\"content\":{\"sides\":[{\"content\":{\"connectorIds\":[\"In3\",\"In4\",\"In2\",\"In5\",\"In1\"]},\"type\":\"ConnectorPlacement.EquallySpacedRectSide\",\"uuid\":\"91d656ef-4f5d-49c3-bf5e-ded947f63a7e\"},{\"content\":{\"connectorIds\":[\"Out1\"],\"side\":\"RIGHT\"},\"type\":\"ConnectorPlacement.EquallySpacedRectSide\",\"uuid\":\"33ea7cbc-c5bc-4b8a-9ce5-c2218895094f\"},{\"content\":{\"connectorIds\":[],\"side\":\"TOP\"},\"type\":\"ConnectorPlacement.EquallySpacedRectSide\",\"uuid\":\"7ad53edd-2f7d-4b13-a1ac-17677a8b969b\"}]},\"type\":\"ConnectorPlacement.EquallySpacedConnector\",\"uuid\":\"c2bfdf98-62c4-4876-963e-3161bc30912a\"}],\"packageUris\":[\"http://schema.mathworks.com/mf0/Connector/R2020b\"],\"version\":\"1.0\"}"
  Clock : Clock
  Stop Simulation : Stop
  Unit Delay : UnitDelay  HasFrameUpgradeWarning=on
  Unit Delay3 : UnitDelay  HasFrameUpgradeWarning=on
  wires:
  Chart/1(doStop) -> Stop Simulation/1
  Clock/1 -> Chart/1(time)
  <TrqCmd>/1 -> Unit Delay/1, Chart/3(trqCmd)
  Unit Delay3/1 -> Chart/5(trq_1)
  <EngTrq>/1 -> Unit Delay3/1, Chart/2(trq)
  Unit Delay/1 -> Chart/4(trqCmd_1)

== system EngineDynamometer/Performance Monitor/Dynamic Logging ==
  LogData : Inport
  Bus Creator : BusCreator  Inputs=9
  Bus Selector : BusSelector  OutputSignals=Torque command (N*m),Measured engine torque (N*m),Engine speed (rpm),BSFC (g/(kW*hr)),Fuel mass flow rate (g/s),Intake port mass flow rate (g/s),Turbocharger shaft speed (rpm),Intake manifold pressure (kPa),Time (s)
  To Workspace : ToWorkspace  VariableName=DynamicDynoSimOut  SampleTime=-1
      settings: Decimation=100
  wires:
  Bus Selector/7 -> Bus Creator/7  "<Turbocharger shaft speed (rpm)>"
  Bus Selector/1 -> Bus Creator/1  "<Torque command (N*m)>"
  Bus Selector/6 -> Bus Creator/6  "<Intake port mass flow rate (g/s)>"
  Bus Selector/4 -> Bus Creator/4  "<BSFC (g/(kW*hr))>"
  Bus Selector/5 -> Bus Creator/5  "<Fuel mass flow rate (g/s)>"
  Bus Selector/3 -> Bus Creator/3  "<Engine speed (rpm)>"
  Bus Selector/2 -> Bus Creator/2  "<Measured engine torque (N*m)>"
  Bus Selector/8 -> Bus Creator/8  "<Intake manifold pressure (kPa)>"
  Bus Selector/9 -> Bus Creator/9  "<Time (s)>"
  Bus Creator/1 -> To Workspace/1
  LogData/1 -> Bus Selector/1  "DynMeasurements"

== system EngineDynamometer/Performance Monitor/Steady State Logging ==
  LogData : Inport
  Trigger : TriggerPort  VariantControl=Variant  PortDimensions=1
  To Workspace : ToWorkspace  VariableName=SteadyDynoSimOut  SampleTime=-1
  wires:
  LogData/1 -> To Workspace/1

== system EngineDynamometer/Performance Monitor/Waitbar ==
  FracComplete : Inport
  Function-Call Generator : FunctionCallGenerator  SampleTime=5
  Function-Call Subsystem : Subsystem  TreatAsAtomicUnit=on
  Rate Transition : RateTransition
  wires:
  Rate Transition/1 -> Function-Call Subsystem/1(FracComplete)
  Function-Call Generator/1 -> Function-Call Subsystem/Trigger
  FracComplete/1 -> Rate Transition/1

== system EngineDynamometer/Dynamometer/Dynamometer Plant/Cooling Fan ==
  FanFlwSpdCmd : Inport
  Bus Selector : BusSelector  OutputSignals=FanFlwSpdCmd
  Cooling Fan Dynamics : TransferFcn  Denominator=[0.4 1]
  FanFlwSpd : Outport  VectorParamsAs1DForOutWhenUnconnected=off
  wires:
  FanFlwSpdCmd/1 -> Bus Selector/1
  Cooling Fan Dynamics/1 -> FanFlwSpd/1
  Bus Selector/1 -> Cooling Fan Dynamics/1  "<FanFlwSpdCmd>"

== system EngineDynamometer/Dynamometer/Dynamometer Plant/Dynamometer Load Motor ==
  DynoCtrl : Inport
  Bus Selector : BusSelector  OutputSignals=EngSpdCmd
  Dyno Dynamics : TransferFcn  Denominator=[0.1 1]
  Signal Specification : SignalSpecification  Unit=rpm
  EngSpd : Outport  VectorParamsAs1DForOutWhenUnconnected=off
  wires:
  Dyno Dynamics/1 -> Signal Specification/1
  DynoCtrl/1 -> Bus Selector/1
  Bus Selector/1 -> Dyno Dynamics/1  "<EngSpdCmd>"
  Signal Specification/1 -> EngSpd/1

== system EngineDynamometer/Dynamometer Control/Open Loop/Open-Loop AFR Control ==
  AfrCmd : Inport
  EngSpd : Inport  Port=2
  TrqCmd : Inport  Port=3
  EstIntkAirMassFlw : Inport  Port=4
  "  " : Product  Inputs=**
  " 1" : Product  Inputs=***///
  Constant : Constant  Value=0
  Fuel Cut : Switch  Criteria=u2 > Threshold  SaturateOnIntegerOverflow=off  InputSameDT=off
  Fuel Flow Rate : Product  Inputs=*/
  Injector Slope mg/ms : Constant  Value=PlntEngSinj
  Saturation : Saturate  UpperLimit=inf  LowerLimit=1
  Saturation1 : Saturate  UpperLimit=inf  LowerLimit=1e-6  ZeroCross=off
  inj per cycle : Constant  Value=PlntEngNCyl
  kg/s to g/s : Gain  Gain=1000
  mg per g : Constant  Value=1000
  rev per cycle : Constant  Value=PlntEngCps
  sec per min : Constant  Value=60
  InjPw : Outport  VectorParamsAs1DForOutWhenUnconnected=off
  wires:
  Saturation1/1 -> Fuel Cut/1
  kg/s to g/s/1 -> Fuel Flow Rate/1
  AfrCmd/1 -> Fuel Flow Rate/2
  EstIntkAirMassFlw/1 -> kg/s to g/s/1
  Fuel Flow Rate/1 -> "  "/1
  rev per cycle/1 -> " 1"/1
  Injector Slope mg/ms/1 -> " 1"/5
  sec per min/1 -> " 1"/3
  EngSpd/1 -> Saturation/1
  mg per g/1 -> " 1"/2
  inj per cycle/1 -> " 1"/4
  " 1"/1 -> "  "/2
  Saturation/1 -> " 1"/6
  "  "/1 -> Saturation1/1
  TrqCmd/1 -> Fuel Cut/2
  Constant/1 -> Fuel Cut/3
  Fuel Cut/1 -> InjPw/1

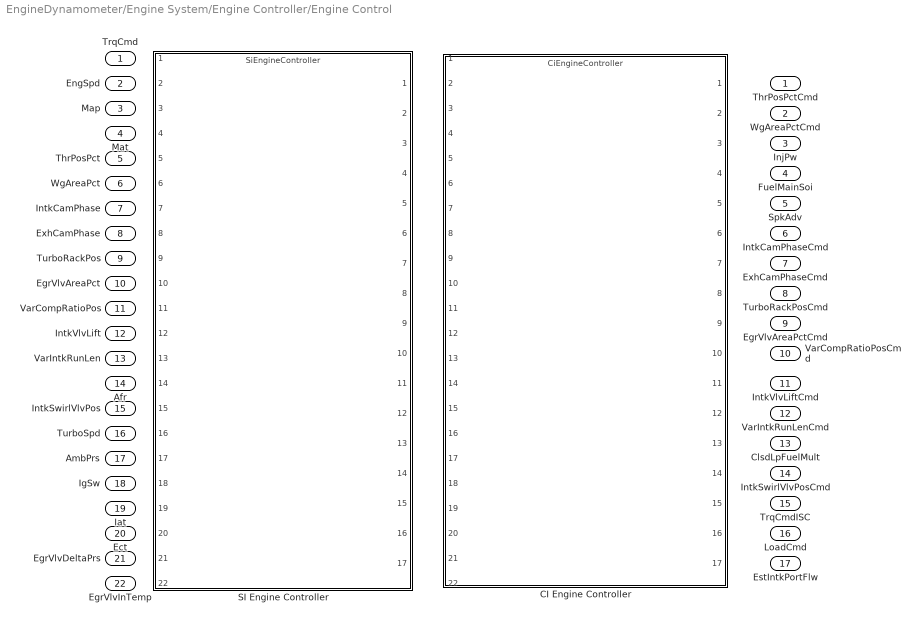
== system EngineDynamometer/Engine System/Engine Controller/Engine Control ==
  TrqCmd : Inport
  EngSpd : Inport  Port=2
  Map : Inport  Port=3
  Mat : Inport  Port=4
  ThrPosPct : Inport  Port=5
  WgAreaPct : Inport  Port=6
  IntkCamPhase : Inport  Port=7
  ExhCamPhase : Inport  Port=8
  TurboRackPos : Inport  Port=9
  EgrVlvAreaPct : Inport  Port=10
  VarCompRatioPos : Inport  Port=11
  IntkVlvLift : Inport  Port=12
  VarIntkRunLen : Inport  Port=13
  Afr : Inport  Port=14
  IntkSwirlVlvPos : Inport  Port=15
  TurboSpd : Inport  Port=16
  AmbPrs : Inport  Port=17
  IgSw : Inport  Port=18
  Iat : Inport  Port=19
  Ect : Inport  Port=20
  EgrVlvDeltaPrs : Inport  Port=21
  EgrVlvInTemp : Inport  Port=22
  CI Engine Controller : ModelReference  ModelNameDialog=CiEngineController.slx  SimulationMode=Normal  VariantControl=CI Engine Controller  ModelReferenceVersion=12.0
  SI Engine Controller : ModelReference  ModelNameDialog=SiEngineController.slx  SimulationMode=Normal  VariantControl=SI Engine Controller  ModelReferenceVersion=11.0
  ThrPosPctCmd : Outport
  WgAreaPctCmd : Outport  Port=2
  InjPw : Outport  Port=3
  FuelMainSoi : Outport  Port=4
  SpkAdv : Outport  Port=5
  IntkCamPhaseCmd : Outport  Port=6
  ExhCamPhaseCmd : Outport  Port=7
  TurboRackPosCmd : Outport  Port=8
  EgrVlvAreaPctCmd : Outport  Port=9
  VarCompRatioPosCmd : Outport  Port=10
  IntkVlvLiftCmd : Outport  Port=11
  VarIntkRunLenCmd : Outport  Port=12
  ClsdLpFuelMult : Outport  Port=13
  IntkSwirlVlvPosCmd : Outport  Port=14
  TrqCmdISC : Outport  Port=15
  LoadCmd : Outport  Port=16
  EstIntkPortFlw : Outport  Port=17

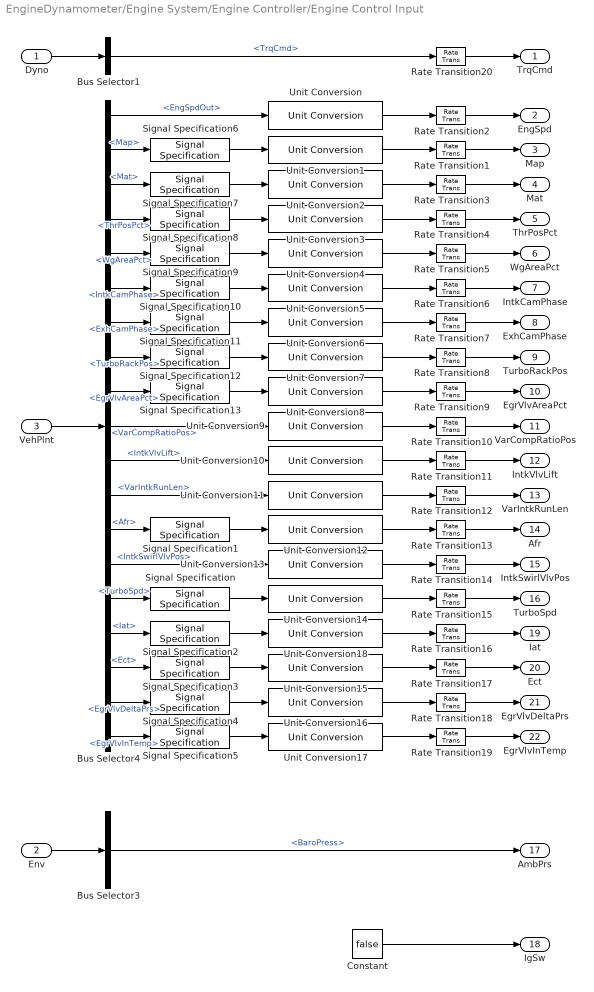
== system EngineDynamometer/Engine System/Engine Controller/Engine Control Input ==
  Dyno : Inport
  Env : Inport  Port=2
  VehPlnt : Inport  Port=3
  Bus Selector1 : BusSelector  OutputSignals=DynoCtrl.TrqCmd
  Bus Selector3 : BusSelector  OutputSignals=BaroPress
  Bus Selector4 : BusSelector  OutputSignals=EngSpdOut,Map,Mat,ThrPosPct,WgAreaPct,IntkCamPhase,ExhCamPhase,TurboRackPos,EgrVlvAreaPct,VarCompRatioPos,IntkVlvLift,VarIntkRunLen,Afr,IntkSwirlVlvPos,TurboSpd,Iat,Ect,EgrVlvDeltaPrs,EgrVlvInTemp
  Constant : Constant  Value=false
  Rate Transition{1..20} (20 alike) : RateTransition
  Signal Specification : SignalSpecification  Unit=rad/sec
  Signal Specification{1,8..9,12..13} (5 alike) : SignalSpecification  Unit=1
  Signal Specification10 : SignalSpecification  Unit=deg
  Signal Specification11 : SignalSpecification  Unit=deg
  Signal Specification{2..3,5,7} (4 alike) : SignalSpecification  Unit=K
  Signal Specification4 : SignalSpecification  Unit=Pa
  Signal Specification6 : SignalSpecification  Unit=Pa
  Unit Conversion{,1..18} (19 alike) : UnitConversion
  TrqCmd : Outport  VectorParamsAs1DForOutWhenUnconnected=off
  EngSpd : Outport  Port=2  VectorParamsAs1DForOutWhenUnconnected=off
  Map : Outport  Port=3  VectorParamsAs1DForOutWhenUnconnected=off
  Mat : Outport  Port=4  VectorParamsAs1DForOutWhenUnconnected=off
  ThrPosPct : Outport  Port=5  VectorParamsAs1DForOutWhenUnconnected=off
  WgAreaPct : Outport  Port=6  VectorParamsAs1DForOutWhenUnconnected=off
  IntkCamPhase : Outport  Port=7  VectorParamsAs1DForOutWhenUnconnected=off
  ExhCamPhase : Outport  Port=8  VectorParamsAs1DForOutWhenUnconnected=off
  TurboRackPos : Outport  Port=9  VectorParamsAs1DForOutWhenUnconnected=off
  EgrVlvAreaPct : Outport  Port=10  VectorParamsAs1DForOutWhenUnconnected=off
  VarCompRatioPos : Outport  Port=11  VectorParamsAs1DForOutWhenUnconnected=off
  IntkVlvLift : Outport  Port=12  VectorParamsAs1DForOutWhenUnconnected=off
  VarIntkRunLen : Outport  Port=13  VectorParamsAs1DForOutWhenUnconnected=off
  Afr : Outport  Port=14  VectorParamsAs1DForOutWhenUnconnected=off
  IntkSwirlVlvPos : Outport  Port=15  VectorParamsAs1DForOutWhenUnconnected=off
  TurboSpd : Outport  Port=16  VectorParamsAs1DForOutWhenUnconnected=off
  AmbPrs : Outport  Port=17  VectorParamsAs1DForOutWhenUnconnected=off
  IgSw : Outport  Port=18  VectorParamsAs1DForOutWhenUnconnected=off
  Iat : Outport  Port=19  VectorParamsAs1DForOutWhenUnconnected=off
  Ect : Outport  Port=20  VectorParamsAs1DForOutWhenUnconnected=off
  EgrVlvDeltaPrs : Outport  Port=21  VectorParamsAs1DForOutWhenUnconnected=off
  EgrVlvInTemp : Outport  Port=22  VectorParamsAs1DForOutWhenUnconnected=off
  wires:
  Unit Conversion13/1 -> Rate Transition14/1
  Unit Conversion11/1 -> Rate Transition12/1
  Unit Conversion8/1 -> Rate Transition9/1
  Unit Conversion9/1 -> Rate Transition10/1
  Unit Conversion10/1 -> Rate Transition11/1
  Unit Conversion7/1 -> Rate Transition8/1
  Unit Conversion5/1 -> Rate Transition6/1
  Unit Conversion6/1 -> Rate Transition7/1
  Unit Conversion4/1 -> Rate Transition5/1
  Unit Conversion3/1 -> Rate Transition4/1
  Unit Conversion2/1 -> Rate Transition3/1
  Unit Conversion1/1 -> Rate Transition1/1
  Unit Conversion/1 -> Rate Transition2/1
  Dyno/1 -> Bus Selector1/1
  Env/1 -> Bus Selector3/1
  VehPlnt/1 -> Bus Selector4/1
  Constant/1 -> IgSw/1
  Unit Conversion15/1 -> Rate Transition17/1
  Unit Conversion17/1 -> Rate Transition19/1
  Unit Conversion16/1 -> Rate Transition18/1
  Unit Conversion18/1 -> Rate Transition16/1
  Bus Selector1/1 -> Rate Transition20/1  "<TrqCmd>"
  Bus Selector4/1 -> Unit Conversion/1  "<EngSpdOut>"
  Bus Selector4/2 -> Signal Specification6/1  "<Map>"
  Bus Selector4/3 -> Signal Specification7/1  "<Mat>"
  Bus Selector4/4 -> Signal Specification8/1  "<ThrPosPct>"
  Bus Selector4/5 -> Signal Specification9/1  "<WgAreaPct>"
  Bus Selector4/6 -> Signal Specification10/1  "<IntkCamPhase>"
  Bus Selector4/7 -> Signal Specification11/1  "<ExhCamPhase>"
  Bus Selector4/8 -> Signal Specification12/1  "<TurboRackPos>"
  Bus Selector4/9 -> Signal Specification13/1  "<EgrVlvAreaPct>"
  Bus Selector4/10 -> Unit Conversion9/1  "<VarCompRatioPos>"
  Bus Selector4/11 -> Unit Conversion10/1  "<IntkVlvLift>"
  Bus Selector4/12 -> Unit Conversion11/1  "<VarIntkRunLen>"
  Bus Selector4/13 -> Signal Specification1/1  "<Afr>"
  Bus Selector4/14 -> Unit Conversion13/1  "<IntkSwirlVlvPos>"
  Bus Selector4/15 -> Signal Specification/1  "<TurboSpd>"
  Bus Selector4/16 -> Signal Specification2/1  "<Iat>"
  Bus Selector4/17 -> Signal Specification3/1  "<Ect>"
  Bus Selector4/18 -> Signal Specification4/1  "<EgrVlvDeltaPrs>"
  Bus Selector4/19 -> Signal Specification5/1  "<EgrVlvInTemp>"
  Bus Selector3/1 -> AmbPrs/1  "<BaroPress>"
  Rate Transition2/1 -> EngSpd/1
  Rate Transition1/1 -> Map/1
  Rate Transition3/1 -> Mat/1
  Rate Transition4/1 -> ThrPosPct/1
  Rate Transition5/1 -> WgAreaPct/1
  Rate Transition6/1 -> IntkCamPhase/1
  Rate Transition7/1 -> ExhCamPhase/1
  Rate Transition8/1 -> TurboRackPos/1
  Rate Transition9/1 -> EgrVlvAreaPct/1
  Rate Transition10/1 -> VarCompRatioPos/1
  Rate Transition11/1 -> IntkVlvLift/1
  Rate Transition12/1 -> VarIntkRunLen/1
  Rate Transition13/1 -> Afr/1
  Rate Transition14/1 -> IntkSwirlVlvPos/1
  Rate Transition15/1 -> TurboSpd/1
  Rate Transition16/1 -> Iat/1
  Rate Transition17/1 -> Ect/1
  Rate Transition18/1 -> EgrVlvDeltaPrs/1
  Rate Transition19/1 -> EgrVlvInTemp/1
  Unit Conversion12/1 -> Rate Transition13/1
  Unit Conversion14/1 -> Rate Transition15/1
  Signal Specification/1 -> Unit Conversion14/1
  Signal Specification1/1 -> Unit Conversion12/1
  Signal Specification2/1 -> Unit Conversion18/1
  Signal Specification3/1 -> Unit Conversion15/1
  Signal Specification4/1 -> Unit Conversion16/1
  Signal Specification5/1 -> Unit Conversion17/1
  Signal Specification6/1 -> Unit Conversion1/1
  Signal Specification7/1 -> Unit Conversion2/1
  Rate Transition20/1 -> TrqCmd/1
  Signal Specification8/1 -> Unit Conversion3/1
  Signal Specification9/1 -> Unit Conversion4/1
  Signal Specification10/1 -> Unit Conversion5/1
  Signal Specification11/1 -> Unit Conversion6/1
  Signal Specification12/1 -> Unit Conversion7/1
  Signal Specification13/1 -> Unit Conversion8/1

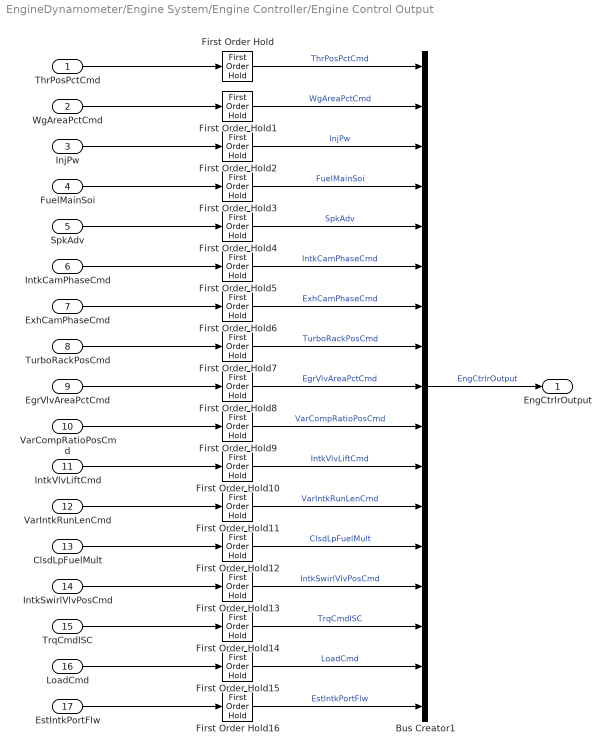
== system EngineDynamometer/Engine System/Engine Controller/Engine Control Output ==
  ThrPosPctCmd : Inport
  WgAreaPctCmd : Inport  Port=2
  InjPw : Inport  Port=3
  FuelMainSoi : Inport  Port=4
  SpkAdv : Inport  Port=5
  IntkCamPhaseCmd : Inport  Port=6
  ExhCamPhaseCmd : Inport  Port=7
  TurboRackPosCmd : Inport  Port=8
  EgrVlvAreaPctCmd : Inport  Port=9
  VarCompRatioPosCmd : Inport  Port=10
  IntkVlvLiftCmd : Inport  Port=11
  VarIntkRunLenCmd : Inport  Port=12
  ClsdLpFuelMult : Inport  Port=13
  IntkSwirlVlvPosCmd : Inport  Port=14
  TrqCmdISC : Inport  Port=15
  LoadCmd : Inport  Port=16
  EstIntkPortFlw : Inport  Port=17
  Bus Creator1 : BusCreator  Inputs=17
  First Order Hold{,1..16} (17 alike) : FirstOrderHold  ErrorTolerance=inf
  EngCtrlrOutput : Outport  VectorParamsAs1DForOutWhenUnconnected=off
  wires:
  VarCompRatioPosCmd/1 -> First Order Hold9/1
  IntkSwirlVlvPosCmd/1 -> First Order Hold13/1
  IntkVlvLiftCmd/1 -> First Order Hold10/1
  VarIntkRunLenCmd/1 -> First Order Hold11/1
  ClsdLpFuelMult/1 -> First Order Hold12/1
  TurboRackPosCmd/1 -> First Order Hold7/1
  TrqCmdISC/1 -> First Order Hold14/1
  ExhCamPhaseCmd/1 -> First Order Hold6/1
  IntkCamPhaseCmd/1 -> First Order Hold5/1
  InjPw/1 -> First Order Hold2/1
  WgAreaPctCmd/1 -> First Order Hold1/1
  EgrVlvAreaPctCmd/1 -> First Order Hold8/1
  LoadCmd/1 -> First Order Hold15/1
  ThrPosPctCmd/1 -> First Order Hold/1
  FuelMainSoi/1 -> First Order Hold3/1
  SpkAdv/1 -> First Order Hold4/1
  EstIntkPortFlw/1 -> First Order Hold16/1
  First Order Hold/1 -> Bus Creator1/1  "ThrPosPctCmd"
  First Order Hold1/1 -> Bus Creator1/2  "WgAreaPctCmd"
  First Order Hold2/1 -> Bus Creator1/3  "InjPw"
  First Order Hold3/1 -> Bus Creator1/4  "FuelMainSoi"
  First Order Hold4/1 -> Bus Creator1/5  "SpkAdv"
  First Order Hold5/1 -> Bus Creator1/6  "IntkCamPhaseCmd"
  Bus Creator1/1 -> EngCtrlrOutput/1  "EngCtrlrOutput"
  First Order Hold6/1 -> Bus Creator1/7  "ExhCamPhaseCmd"
  First Order Hold7/1 -> Bus Creator1/8  "TurboRackPosCmd"
  First Order Hold8/1 -> Bus Creator1/9  "EgrVlvAreaPctCmd"
  First Order Hold9/1 -> Bus Creator1/10  "VarCompRatioPosCmd"
  First Order Hold10/1 -> Bus Creator1/11  "IntkVlvLiftCmd"
  First Order Hold11/1 -> Bus Creator1/12  "VarIntkRunLenCmd"
  First Order Hold12/1 -> Bus Creator1/13  "ClsdLpFuelMult"
  First Order Hold13/1 -> Bus Creator1/14  "IntkSwirlVlvPosCmd"
  First Order Hold14/1 -> Bus Creator1/15  "TrqCmdISC"
  First Order Hold15/1 -> Bus Creator1/16  "LoadCmd"
  First Order Hold16/1 -> Bus Creator1/17  "EstIntkPortFlw"

== system EngineDynamometer/Engine System/Engine Plant/Engine ==
  Env : Inport
  EngSpd : Inport  Port=2
  Veh : Inport  Port=3
  Cntrl : Inport  Port=4
  CI Engine : Subsystem  VariantControl=CI Engine  ReferencedSubsystem=CiEngine
  CI Mapped Engine : Subsystem  VariantControl=CI Mapped Engine  ReferencedSubsystem=CiMappedEngine
  SI DL Engine : Subsystem  VariantControl=SI DL Engine  ReferencedSubsystem=SiDLEngine
  SI Engine : Subsystem  VariantControl=SI Engine  ReferencedSubsystem=SiEngine
  SI Mapped Engine : Subsystem  VariantControl=SI Mapped Engine  ReferencedSubsystem=SiMappedEngine
  Simple Engine : Subsystem  VariantControl=Simple Engine  ReferencedSubsystem=SimpleEngine
  EngFdbk : Outport

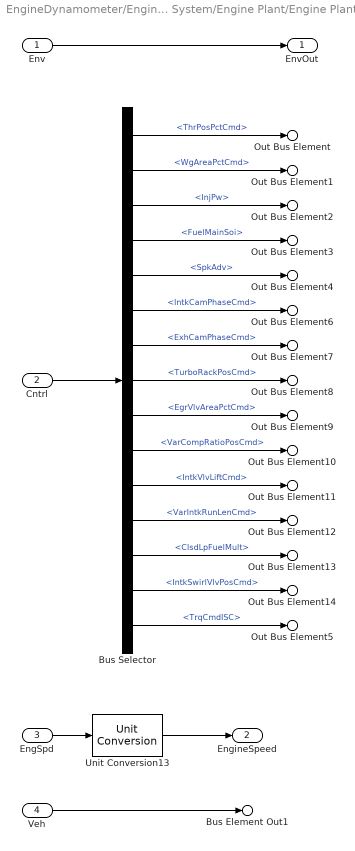
== system EngineDynamometer/Engine System/Engine Plant/Engine Plant Input ==
  Env : Inport
  Cntrl : Inport  Port=2
  EngSpd : Inport  Port=3
  Veh : Inport  Port=4
  Bus Selector : BusSelector  OutputSignals=ThrPosPctCmd,WgAreaPctCmd,InjPw,FuelMainSoi,SpkAdv,IntkCamPhaseCmd,ExhCamPhaseCmd,TurboRackPosCmd,EgrVlvAreaPctCmd,VarCompRatioPosCmd,IntkVlvLiftCmd,VarIntkRunLenCmd,ClsdLpFuelMult,IntkSwirlVlvPosCmd,TrqCmdISC
  Unit Conversion13 : UnitConversion
  EnvOut : Outport
  EngineSpeed : Outport  Port=2
  Bus Element Out1 : Outport  Port=3  PortName=Dyno  Element=BdyFrm.Cg.Vel.xdot
  Out Bus Element : Outport  Port=4  PortName=Ctrl  Element=Engine.ThrPosPctCmd
  Out Bus Element1 : Outport  Port=4  PortName=Ctrl  Element=Engine.WgAreaPctCmd
  Out Bus Element2 : Outport  Port=4  PortName=Ctrl  Element=Engine.InjPw
  Out Bus Element3 : Outport  Port=4  PortName=Ctrl  Element=Engine.FuelMainSoi
  Out Bus Element4 : Outport  Port=4  PortName=Ctrl  Element=Engine.SpkAdv
  Out Bus Element6 : Outport  Port=4  PortName=Ctrl  Element=Engine.IntkCamPhaseCmd
  Out Bus Element7 : Outport  Port=4  PortName=Ctrl  Element=Engine.ExhCamPhaseCmd
  Out Bus Element8 : Outport  Port=4  PortName=Ctrl  Element=Engine.TurboRackPosCmd
  Out Bus Element9 : Outport  Port=4  PortName=Ctrl  Element=Engine.EgrVlvAreaPctCmd
  Out Bus Element10 : Outport  Port=4  PortName=Ctrl  Element=Engine.VarCompRatioPosCmd
  Out Bus Element11 : Outport  Port=4  PortName=Ctrl  Element=Engine.IntkVlvLiftCmd
  Out Bus Element12 : Outport  Port=4  PortName=Ctrl  Element=Engine.VarIntkRunLenCmd
  Out Bus Element13 : Outport  Port=4  PortName=Ctrl  Element=Engine.ClsdLpFuelMult
  Out Bus Element14 : Outport  Port=4  PortName=Ctrl  Element=Engine.IntkSwirlVlvPosCmd
  Out Bus Element5 : Outport  Port=4  PortName=Ctrl  Element=Engine.TrqCmd
  wires:
  Env/1 -> EnvOut/1
  EngSpd/1 -> Unit Conversion13/1
  Unit Conversion13/1 -> EngineSpeed/1
  Veh/1 -> Bus Element Out1/1
  Bus Selector/1 -> Out Bus Element/1  "<ThrPosPctCmd>"
  Bus Selector/7 -> Out Bus Element7/1  "<ExhCamPhaseCmd>"
  Bus Selector/6 -> Out Bus Element6/1  "<IntkCamPhaseCmd>"
  Cntrl/1 -> Bus Selector/1
  Bus Selector/13 -> Out Bus Element13/1  "<ClsdLpFuelMult>"
  Bus Selector/5 -> Out Bus Element4/1  "<SpkAdv>"
  Bus Selector/12 -> Out Bus Element12/1  "<VarIntkRunLenCmd>"
  Bus Selector/11 -> Out Bus Element11/1  "<IntkVlvLiftCmd>"
  Bus Selector/3 -> Out Bus Element2/1  "<InjPw>"
  Bus Selector/4 -> Out Bus Element3/1  "<FuelMainSoi>"
  Bus Selector/10 -> Out Bus Element10/1  "<VarCompRatioPosCmd>"
  Bus Selector/8 -> Out Bus Element8/1  "<TurboRackPosCmd>"
  Bus Selector/2 -> Out Bus Element1/1  "<WgAreaPctCmd>"
  Bus Selector/9 -> Out Bus Element9/1  "<EgrVlvAreaPctCmd>"
  Bus Selector/15 -> Out Bus Element5/1  "<TrqCmdISC>"
  Bus Selector/14 -> Out Bus Element14/1  "<IntkSwirlVlvPosCmd>"

== system EngineDynamometer/Performance Monitor/Waitbar/Function-Call Subsystem ==
  FracComplete : Inport
  function : TriggerPort  TriggerType=function-call  VariantControl=Variant
  Waitbar : MATLAB Function  TreatAsAtomicUnit=on
  wires:
  FracComplete/1 -> Waitbar/1(FracComplete)

== stateflow chart EngineDynamometer/Dynamometer Control/Steady State/Select Operating Point ==
  settings: executeAtInitialization=1
  state SetInitialPoint
    en:
    EngSpd = 0;
    TrqCmd = 0;
  state Startup
    en:
    EngSpd = EngSpdCmdPts(Index);
    TrqCmd = TrqCmdPts(Index);
    TotNumPoints = min(numel(EngSpdCmdPts), numel(TrqCmdPts));
  state LogData
    ex:
    LogDataTrigger = true;
  state WaitForSteadyState
    en:
    FracComplete = Index/TotNumPoints;
    LogDataTrigger = false;
  state SetNewValue
    en:
    Index = Index + 1;
    EngSpd = EngSpdCmdPts(Index);
    TrqCmd = TrqCmdPts(Index);
  state Stop
    en:
    FracComplete = 1;
    StopCmd = true;
  (default) -> SetInitialPoint : {
      | Index = 1;
      | StopCmd = false;
      | LogDataTrigger = false;
      | FracComplete = 0;
      | }
  SetInitialPoint -> Startup
  Startup -> WaitForSteadyState : after(5,sec)
  WaitForSteadyState -> LogData [order 2] : after(SteadyStateWaitLimit, sec)
  LogData -> (junction 73) : after(0.01, sec)
  (junction 73) -> SetNewValue [order 1] : [Index < numel(EngSpdCmdPts) || Index < numel(TrqCmdPts)]
  (junction 73) -> Stop [order 2]
  WaitForSteadyState -> LogData [order 1] : [SteadyStateFlag]
  SetNewValue -> WaitForSteadyState [order 1] : after(0.1,sec)[~SteadyStateFlag]
  SetNewValue -> WaitForSteadyState [order 2] : after(1.5,sec)
  data: SteadyStateFlag input; SteadyStateWaitLimit input; EngSpd output; EngSpdCmdPts input; TrqCmdPts input; TrqCmd output; Index local; LogDataTrigger output; StopCmd output; FracComplete output; TotNumPoints local
